simulink model "SPI_Test"  (R2015b)
settings: Solver=FixedStepDiscrete  StartTime=0.0  StopTime=10.0  RelTol=1e-3
libraries: SPI_Lib x1, STM32_Config_Lib x1
settings Model: Creator=brunj  LastModifiedBy=reynaudp
settings DataIOCC: SaveFormat=Array
settings OptimizationCC: OptimizeModelRefInitCode=on  LifeSpan=1
settings DebuggingCC: UnderspecifiedInitializationDetection=Classic  MergeDetectMultiDrivingBlocksExec=none  SolverPrmCheckMsg=warning
settings HardwareCC: ProdBitPerPointer=32  ProdLargestAtomicInteger=Integer  ProdWordSize=32  ProdHWDeviceType=STMicroelectronics->STM32 32-bit Cortex-M
settings RTWCC: SystemTargetFile=stm32.tlc  TemplateMakefile=stm32.tmf  Description=stm32 (Embedded Target)  GenerateReport=on
settings CodeAppCC: IgnoreCustomStorageClasses=off  MaxIdLength=64  CustomSymbolStrType=$N$R$M  SimulinkBlockComments=off
settings STFCustomTargetCC: CodeReplacementLibrary=ARM CMSIS SIN COS  ParMdlRefBuildCompliant=on  ConcurrentExecutionCompliant=off  IncludeMdlTerminateFcn=off  GeneratePreprocessorConditionals=Use local settings  CombineOutputUpdateFcns=on  ERTCustomFileBanners=on  SupportContinuousTime=off  MATLABClassNameForMDSCustomization=Simulink.SoftwareTarget.ERTCustomization  CPPClassGenCompliant=off  GRTInterface=off  SystemTargetFile=stm32.tlc
settings ERTTargetCC: CodeReplacementLibrary=ARM CMSIS SIN COS  CompOptLevelCompliant=off  ConcurrentExecutionCompliant=off  IncludeMdlTerminateFcn=off  ERTFirstTimeCompliant=off  SupportNonInlinedSFcns=on  ModelStepFunctionPrototypeControlCompliant=off  CPPClassGenCompliant=off  UseToolchainInfoCompliant=off  ERTSrcFileBannerTemplate=sourceFileTemplate.cgt  ERTHdrFileBannerTemplate=sourceFileTemplate.cgt  ERTDataSrcFileTemplate=sourceFileTemplate.cgt  ERTDataHdrFileTemplate=sourceFileTemplate.cgt  ERTCustomFileTemplate=customRoutineProcess.tlc
settings ConfigComp: CovModelRefEnable=Off  CovSFcnEnable=off

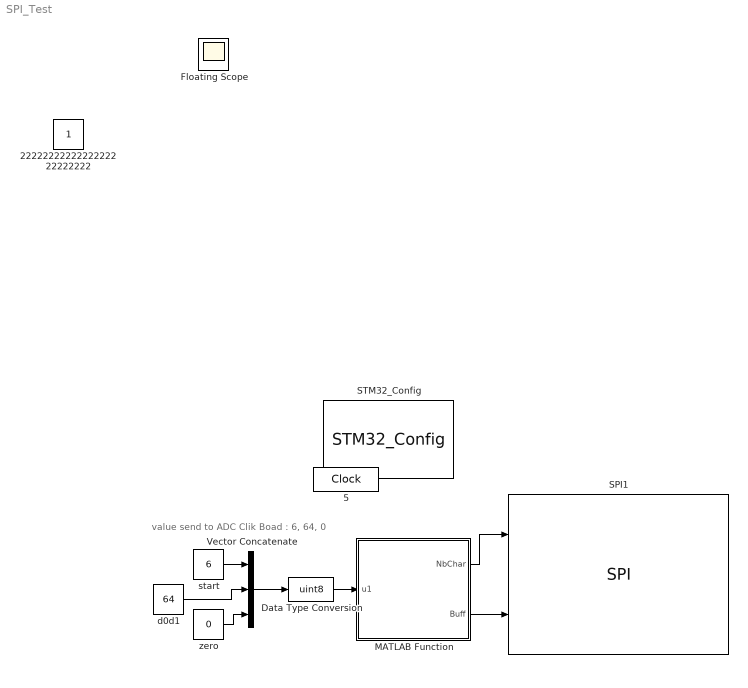
== system SPI_Test ==
  note: value send to ADC Clik Boad : 6, 64, 0
  Data Type Conversion : DataTypeConversion  OutDataTypeStr=uint8
  MATLAB Function : MATLAB Function  TreatAsAtomicUnit=on
  SPI1 : SPI_Lib/SPI  SPIx=SPI1  Device_Mode=MASTER  Type_SPI=Full_Duplex  SPI_Mode=POLLING  handler=hspi1  Buffer_Size_Rcv=5  Buffer_Size_Send=5  NbSPI=2  Nb_bits_transmission=8  Timeout=-1  TimeoutValue=0.001  NSS=off  Error=off  CallBack=off  Transmission=off
  STM32_Config : STM32_Config_Lib/STM32_Config  Priority=0  Project_Path=.\  Config_File=SPI_Test.ioc  MCU_Name=STM32L053R8Tx
  Vector Concatenate : Concatenate  NumInputs=3
  d0d1 : Constant  Value=64  OutDataTypeStr=uint8
  start : Constant  Value=6  OutDataTypeStr=uint8
  zero : Constant  Value=0  OutDataTypeStr=uint8
  2222222222222222222222222 : Constant  IOType=siggen
  5 : DigitalClock  IOType=siggen
  Floating Scope : Scope
  wires:
  start/1 -> Vector Concatenate/1
  Vector Concatenate/1 -> Data Type Conversion/1
  Data Type Conversion/1 -> MATLAB Function/1(u1)
  d0d1/1 -> Vector Concatenate/2
  zero/1 -> Vector Concatenate/3
  MATLAB Function/1(NbChar) -> SPI1/1
  MATLAB Function/2(Buff) -> SPI1/2

== matlab function SPI_Test/MATLAB Function ==
  data: u1 input; NbChar output; Buff output
function [NbChar, Buff]     = generateBuff(u1)
    if coder.target('Sfun')
        % Executing in MATLAB, Buff is null
        Buff = uint32(0);
        NbChar = uint16(0);
    else
        % Executing in the generated code. 
      Buff = uint32(0);
      Buff = coder.ceval('getBuffPtr_SPI',uint8(u1));
      [nbChar,~] = size(u1);
      NbChar = uint16(nbChar);
         
    end
end
%Buff = uint32(y);
%%Buff = [buffer(1:4), tmp, 13, 10, 0];
